simulink model "SatStates"  (R2020b)
settings: Solver=VariableStepAuto  StartTime=0.0  StopTime=3*24*3600  RelTol=1e-9
settings Model: Creator=daniel  LastModifiedBy=daniel

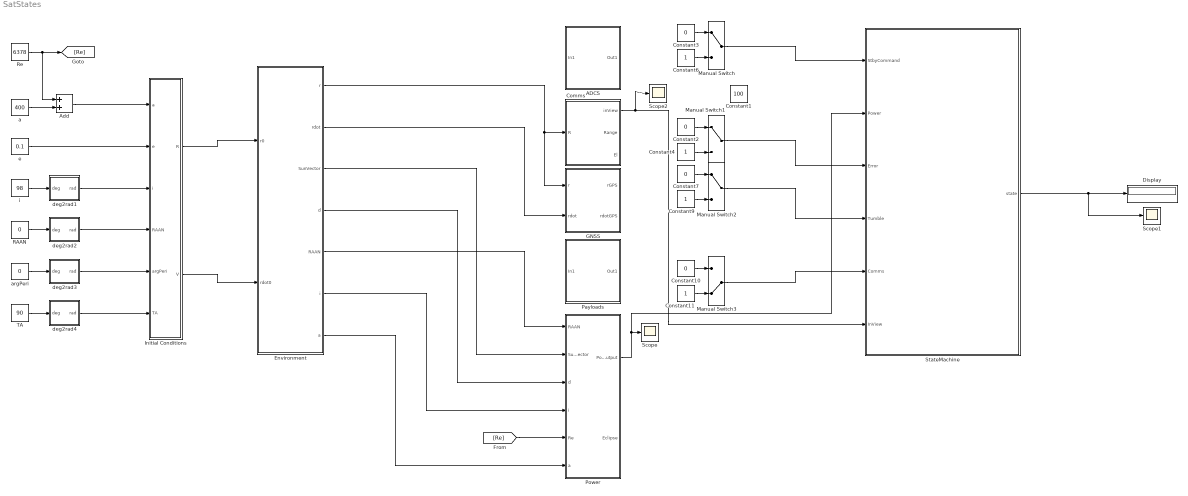
== system SatStates ==
  " Initial Conditions" : MATLAB Function  TreatAsAtomicUnit=on
  ADCS : Subsystem
  Add : Sum
  Comms : Subsystem
  Constant1 : Constant  Value=100
  Constant{2..3,7,10} (4 alike) : Constant  Value=0
  Constant{4,6,9,11} (4 alike) : Constant
  Display : Display
  Environment : Subsystem
  GNSS : Subsystem
  Manual Switch : ManualSwitch
  Manual Switch1 : ManualSwitch
  Manual Switch2 : ManualSwitch
  Manual Switch3 : ManualSwitch  CurrentSetting=0
  Payloads : Subsystem
  Power : Subsystem
  RAAN : Constant  Value=0
  Re : Constant  Value=6378
  Scope : Scope
  Scope1 : Scope
  Scope2 : Scope
  StateMachine : Stateflow chart  TreatAsAtomicUnit=on
  TA : Constant  Value=90
  a : Constant  Value=400
  argPeri : Constant  Value=0
  deg2rad1 : MATLAB Function  TreatAsAtomicUnit=on
  deg2rad2 : MATLAB Function  TreatAsAtomicUnit=on
  deg2rad3 : MATLAB Function  TreatAsAtomicUnit=on
  deg2rad4 : MATLAB Function  TreatAsAtomicUnit=on
  e : Constant  Value=0.1
  i : Constant  Value=98
  wires:
  Manual Switch/1 -> StateMachine/1(StbyCommand)
  Manual Switch3/1 -> StateMachine/5(Comms)
  StateMachine/1(state) -> Scope1/1, Display/1
  Constant3/1 -> Manual Switch/1
  Constant6/1 -> Manual Switch/2
  Constant4/1 -> Manual Switch1/2
  Constant2/1 -> Manual Switch1/1
  Manual Switch1/1 -> StateMachine/3(Error)
  Manual Switch2/1 -> StateMachine/4(Tumble)
  Constant7/1 -> Manual Switch2/1
  Constant9/1 -> Manual Switch2/2
  Constant11/1 -> Manual Switch3/2
  Constant10/1 -> Manual Switch3/1
  Environment/1(r) -> GNSS/1(r), Comms/1(R)
  Environment/2(rdot) -> GNSS/2(rdot)
  " Initial Conditions"/1(R) -> Environment/1(r0)
  " Initial Conditions"/2(V) -> Environment/2(rdot0)
  Environment/5(RAAN) -> Power/1(RAAN)
  Environment/4(d) -> Power/3(d)
  Environment/3(SunVector) -> Power/2(SunVector)
  Environment/6(i) -> Power/4(i)
  Environment/7(a) -> Power/6(a)
  Power/1(Power Output) -> StateMachine/2(Power), Scope/1
  TA/1 -> deg2rad4/1(deg)
  argPeri/1 -> deg2rad3/1(deg)
  RAAN/1 -> deg2rad2/1(deg)
  i/1 -> deg2rad1/1(deg)
  a/1 -> Add/2
  Re/1 -> [Re], Add/1
  Add/1 -> " Initial Conditions"/1(a)
  e/1 -> " Initial Conditions"/2(e)
  deg2rad1/1(rad) -> " Initial Conditions"/3(i)
  deg2rad2/1(rad) -> " Initial Conditions"/4(RAAN)
  deg2rad3/1(rad) -> " Initial Conditions"/5(argPeri)
  deg2rad4/1(rad) -> " Initial Conditions"/6(TA)
  [Re] -> Power/5(Re)
  Comms/1(inView) -> Scope2/1, StateMachine/6(InView)

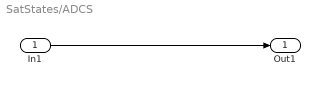
== system SatStates/ADCS ==
  In1 : Inport
  Out1 : Outport
  wires:
  In1/1 -> Out1/1

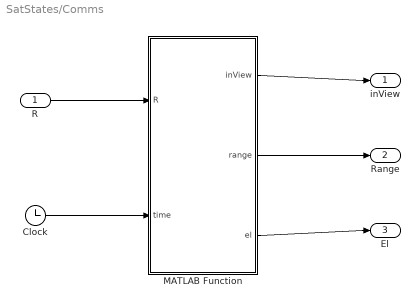
== system SatStates/Comms ==
  R : Inport
  Clock : Clock
  MATLAB Function : MATLAB Function  TreatAsAtomicUnit=on
  inView : Outport
  Range : Outport  Port=2
  El : Outport  Port=3
  wires:
  R/1 -> MATLAB Function/1(R)
  Clock/1 -> MATLAB Function/2(time)
  MATLAB Function/1(inView) -> inView/1
  MATLAB Function/2(range) -> Range/1
  MATLAB Function/3(el) -> El/1

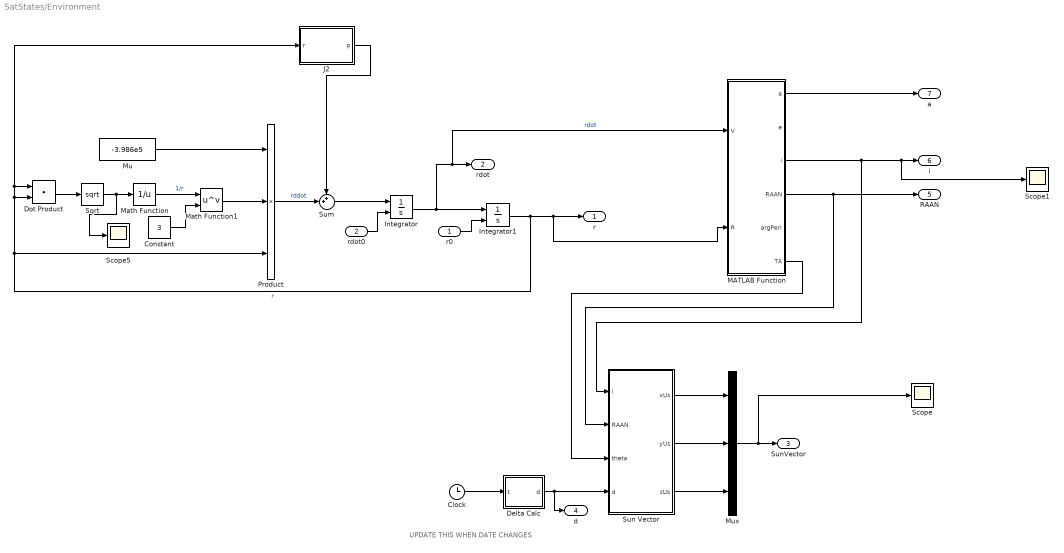
== system SatStates/Environment ==
  note: UPDATE THIS WHEN DATE CHANGES
  r0 : Inport
  rdot0 : Inport  Port=2
  Clock : Clock
  Constant : Constant  Value=3
  Delta Calc : MATLAB Function  TreatAsAtomicUnit=on
  Dot Product : DotProduct  InputSameDT=on  OutDataTypeStr=Inherit: Inherit via internal rule
  Integrator : Integrator  InitialConditionSource=external
  Integrator1 : Integrator  InitialConditionSource=external
  J2 : MATLAB Function  TreatAsAtomicUnit=on
  MATLAB Function : MATLAB Function  TreatAsAtomicUnit=on
  Math Function : Math  Operator=reciprocal  SaturateOnIntegerOverflow=on
  Math Function1 : Math  Operator=pow  SaturateOnIntegerOverflow=on
  Mu : Constant  Value=-3.986e5
  Mux : Mux  Inputs=3
  Product : Product  Inputs=3
  Scope : Scope
  Scope1 : Scope
  Scope5 : Scope
  Sqrt : Sqrt  SaturateOnIntegerOverflow=on
  Sum : Sum  Inputs=++|
  Sun Vector : MATLAB Function  TreatAsAtomicUnit=on
  r : Outport
  rdot : Outport  Port=2
  SunVector : Outport  Port=3  VectorParamsAs1DForOutWhenUnconnected=off
  d : Outport  Port=4  VectorParamsAs1DForOutWhenUnconnected=off
  RAAN : Outport  Port=5  VectorParamsAs1DForOutWhenUnconnected=off
  i : Outport  Port=6  VectorParamsAs1DForOutWhenUnconnected=off
  a : Outport  Port=7  VectorParamsAs1DForOutWhenUnconnected=off
  wires:
  Integrator1/1 -> Product/3, Dot Product/1, J2/1(r), Dot Product/2, r/1, MATLAB Function/2(R)  "r"
  Math Function/1 -> Math Function1/1  "1/r"
  Mu/1 -> Product/1
  Integrator/1 -> MATLAB Function/1(V), rdot/1, Integrator1/1  "rdot"
  rdot0/1 -> Integrator/2
  r0/1 -> Integrator1/2
  Mux/1 -> Scope/1, SunVector/1
  Sun Vector/1(xUs) -> Mux/1
  Sun Vector/2(yUs) -> Mux/2
  Sun Vector/3(zUs) -> Mux/3
  MATLAB Function/3(i) -> Scope1/1, i/1, Sun Vector/1(i)
  MATLAB Function/4(RAAN) -> Sun Vector/2(RAAN), RAAN/1
  MATLAB Function/6(TA) -> Sun Vector/3(theta)
  Delta Calc/1(d) -> Sun Vector/4(d), d/1
  Clock/1 -> Delta Calc/1(t)
  Product/1 -> Sum/2  "rddot"
  Sum/1 -> Integrator/1
  Math Function1/1 -> Product/2
  Constant/1 -> Math Function1/2
  Sqrt/1 -> Scope5/1, Math Function/1
  Dot Product/1 -> Sqrt/1
  J2/1(p) -> Sum/1
  MATLAB Function/1(a) -> a/1

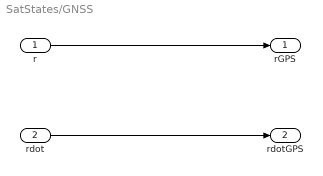
== system SatStates/GNSS ==
  r : Inport
  rdot : Inport  Port=2
  rGPS : Outport
  rdotGPS : Outport  Port=2
  wires:
  r/1 -> rGPS/1
  rdot/1 -> rdotGPS/1

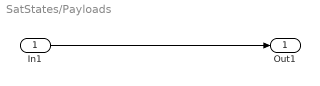
== system SatStates/Payloads ==
  In1 : Inport
  Out1 : Outport
  wires:
  In1/1 -> Out1/1

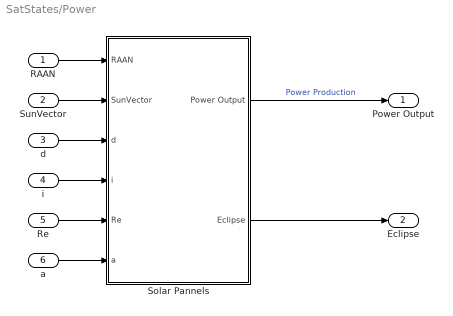
== system SatStates/Power ==
  RAAN : Inport
  SunVector : Inport  Port=2
  d : Inport  Port=3
  i : Inport  Port=4
  Re : Inport  Port=5
  a : Inport  Port=6
  Solar Pannels : Subsystem
  Power Output : Outport
  Eclipse : Outport  Port=2
  wires:
  RAAN/1 -> Solar Pannels/1(RAAN)
  SunVector/1 -> Solar Pannels/2(SunVector)
  d/1 -> Solar Pannels/3(d)
  i/1 -> Solar Pannels/4(i)
  Re/1 -> Solar Pannels/5(Re)
  a/1 -> Solar Pannels/6(a)
  Solar Pannels/1(Power Output) -> Power Output/1  "Power Production"
  Solar Pannels/2(Eclipse) -> Eclipse/1

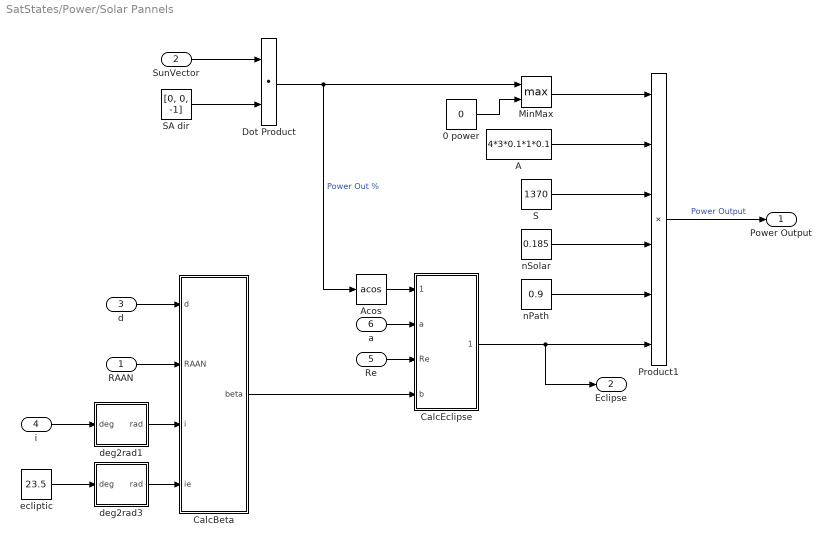
== system SatStates/Power/Solar Pannels ==
  RAAN : Inport
  SunVector : Inport  Port=2
  d : Inport  Port=3
  i : Inport  Port=4
  Re : Inport  Port=5
  a : Inport  Port=6
  0 power : Constant  Value=0
  A : Constant  Value=4*3*0.1*1*0.1
  Acos : Trigonometry  Operator=acos
  CalcBeta : MATLAB Function  TreatAsAtomicUnit=on
  CalcEclipse : MATLAB Function  TreatAsAtomicUnit=on
  Dot Product : DotProduct  InputSameDT=on  OutDataTypeStr=Inherit: Inherit via internal rule
  MinMax : MinMax  Function=max  Inputs=2
  Product1 : Product  Inputs=6
  S : Constant  Value=1370
  SA dir : Constant  Value=[0, 0, -1]
  deg2rad1 : MATLAB Function  TreatAsAtomicUnit=on
  deg2rad3 : MATLAB Function  TreatAsAtomicUnit=on
  ecliptic : Constant  Value=23.5
  nPath : Constant  Value=0.9
  nSolar : Constant  Value=0.185
  Power Output : Outport  VectorParamsAs1DForOutWhenUnconnected=off
  Eclipse : Outport  Port=2  VectorParamsAs1DForOutWhenUnconnected=off
  wires:
  0 power/1 -> MinMax/2
  deg2rad1/1(rad) -> CalcBeta/3(i)
  nSolar/1 -> Product1/4
  CalcEclipse/1(eclipse) -> Product1/6, Eclipse/1
  Product1/1 -> Power Output/1  "Power Output"
  MinMax/1 -> Product1/1
  S/1 -> Product1/3
  Acos/1 -> CalcEclipse/1(sunAng)
  ecliptic/1 -> deg2rad3/1(deg)
  Re/1 -> CalcEclipse/3(Re)
  nPath/1 -> Product1/5
  Dot Product/1 -> MinMax/1, Acos/1  "Power Out %"
  SA dir/1 -> Dot Product/2
  d/1 -> CalcBeta/1(d)
  A/1 -> Product1/2
  a/1 -> CalcEclipse/2(a)
  CalcBeta/1(beta) -> CalcEclipse/4(b)
  deg2rad3/1(rad) -> CalcBeta/4(ie)
  RAAN/1 -> CalcBeta/2(RAAN)
  i/1 -> deg2rad1/1(deg)
  SunVector/1 -> Dot Product/1

== stateflow chart SatStates/StateMachine ==
  state DeviceLogic [parallel]
    settings: executionOrder=1
    note: States:
        | 0 -> Deploy
        | 1 -> Tumble/Recovery
        | 2 -> Normal Operations
        | 3 -> Standby
        | 4 -> Error
        | 5 -> Lower Power
        | 6 -> Ground Station Overpass
    state Standby
      entry: state=3
    state NormalOps
      entry: state=2;
    state GSOverpass
      entry: state=6;
    state TumbleRecovery
      entry: state=1;
    state Deploy
      entry: state=0;
    note: Note: Deploy should have own Error handling or some other way to go back to deploy after error
    state LowPower
      entry: state=5;
    state Error
      entry: state=4;
    NormalOps -> Standby [order 3] : [StbyCommand && after(5, sec)]
    Standby -> NormalOps : [~StbyCommand || after(15, sec)]
    (default) -> Deploy
    TumbleRecovery -> NormalOps [order 2] : [~Tumble]
    NormalOps -> GSOverpass [order 2] : [InView]
    Deploy -> TumbleRecovery : [after(20, sec)]
    NormalOps -> TumbleRecovery [order 5] : [Tumble]
    GSOverpass -> NormalOps [order 2] : [~InView]
    GSOverpass -> Error [order 1] : [Error || ~Comms]
    Error -> TumbleRecovery : [~Error && Comms]
    TumbleRecovery -> Error [order 1] : [Error || ~Comms]
    LowPower -> TumbleRecovery [order 2] : [Power > 10]
    NormalOps -> Error [order 1] : [Error || ~Comms]
    NormalOps -> LowPower [order 4] : [Power < 5]
    LowPower -> Error [order 1] : [Error || ~Comms]
  state PayloadLogic [parallel]
    settings: executionOrder=2
    state On
    state Off
    (default) -> Off
    Off -> On : [isPayloadOn(state)]
    On -> Off : [~isPayloadOn(state)]
  state payloadState=isPayloadOn(var) [function]
    (default) -> (junction 65)
    (junction 65) -> (junction 66) [order 1] : [var==2]
    (junction 65) -> (junction 67) [order 2] : {payloadState = 0;}
    (junction 66) -> (junction 68) : {payloadState = 1;}
    (junction 68) -> (junction 67)
    (junction 67) -> (junction 69)
  data: var function_input; payloadState function_output; StbyCommand input; Power input; Error input; Tumble input; Comms input; state output; InView input

== matlab function SatStates/ Initial Conditions ==
  data: R output; V output; a input; e input; i input; RAAN input; argPeri input; TA input
function [R, V] = fcn(a, e, i, RAAN, argPeri, TA)

mu = 3.986e5;

OE = [sqrt(mu*a*(1-e^2)); e; i; RAAN; argPeri; TA];

[R, V] = OE2SV(mu, OE);

== matlab function SatStates/deg2rad1 ==
  data: deg input; rad output
function rad = fcn(deg)

rad = deg2rad(deg)

== matlab function SatStates/deg2rad2 ==
  data: deg input; rad output
function rad = fcn(deg)

rad = deg2rad(deg)

== matlab function SatStates/Environment/Sun Vector ==
  data: i input; xUs output; RAAN input; theta input; yUs output; zUs output; d input
function [xUs, yUs, zUs] = fcn(i, RAAN, theta, d)
   
   e = deg2rad(23.5);
   
   Sec = [cos(d); sin(d); 0];
   
   Aeceq = [1 0 0; 0 cos(e) -sin(e); 0 sin(e) cos(e)];
   Aeqan = [cos(RAAN) sin(RAAN) 0; -sin(RAAN) cos(RAAN) 0; 0 0 1];
   Aanop = [1 0 0; 0 cos(i) sin(i); 0 -sin(i) cos(i)];
   Aopso = [cos(theta) sin(theta) 0; -sin(theta) cos(theta) 0; 0 0 1];
   AsoB = [0 1 0; -1 0 0; 0 0 1];
   ABLVLH = [1 0 0; 0 0 -1; 0 1 0];
   
   uSLVLH = ABLVLH*AsoB*Aopso*Aanop*Aeqan*Aeceq*Sec;
   
   xUs = uSLVLH(1);
   yUs = uSLVLH(2);
   zUs = uSLVLH(3);
end

== matlab function SatStates/Environment/Delta Calc ==
  data: t input; d output
function d = fcn(t)

% Date of the Sim
%        Day        Min      Hour
const = 0*3600*24 + 0*60 + 0*3600;
deltaT = const + t;
w = 2*pi/(365.25*24*3600);
d = w*deltaT;

== matlab function SatStates/Power/Solar Pannels/CalcEclipse ==
  data: sunAng input; eclipse output; a input; Re input; b input
function eclipse = fcn(sunAng, a, Re, b)

ang = abs(pi - sunAng);

alph = acos(sqrt(a^2 - Re^2)/(a*cos(b)));

if ang < alph
    eclipse = 0;
else
    eclipse = 1;
end

== matlab function SatStates/Power/Solar Pannels/CalcBeta ==
  data: d input; beta output; RAAN input; i input; ie input
function beta = fcn(d, RAAN, i, ie)

beta = asin(cos(d)*sin(RAAN)*sin(i) - sin(d)*cos(ie)*cos(RAAN)*sin(i) -...
    sin(d)*sin(ie)*cos(i));

== matlab function SatStates/Power/Solar Pannels/deg2rad3 ==
  data: deg input; rad output
function rad = fcn(deg)

rad = deg2rad(deg)

== matlab function SatStates/Power/Solar Pannels/deg2rad1 ==
  data: deg input; rad output
function rad = fcn(deg)

rad = deg2rad(deg)

== matlab function SatStates/deg2rad3 ==
  data: deg input; rad output
function rad = fcn(deg)

rad = deg2rad(deg)

== matlab function SatStates/deg2rad4 ==
  data: deg input; rad output
function rad = fcn(deg)

rad = deg2rad(deg)

== matlab function SatStates/Comms/MATLAB Function ==
  data: R input; inView output; time input; range output; el output
function [inView, range, el] = fcn(R, time)

GS = [deg2rad(39.96); deg2rad(-95.25); 3.6];

[inView, range, el] = GS_View(GS, R, time);

== matlab function SatStates/Environment/J2 ==
  data: r input; p output
function p = fcn(r)

rr = norm(r);

Re = 6378;
J2 = 1.082626638e-3;
mu = 3.986e5;

p = 3/2*J2*mu*Re^2/rr^4*[r(1)/rr*(5*r(3)^2/rr^2 - 1); r(2)/rr*(5*r(3)^2/rr^2 - 1); r(3)/rr*(5*r(3)^2/rr^2 - 3)];

== matlab function SatStates/Environment/MATLAB Function ==
  data: V input; a output; R input; e output; i output; RAAN output; argPeri output; TA output
function [a, e, i, RAAN, argPeri, TA] = fcn(V, R)


OE = SV2OE(3.986e5, R, V);

a = OE(7);
e = OE(2);
i = OE(3);
RAAN = OE(4);
argPeri = OE(5);
TA = OE(6);
